simulink model "sim_2dof"  (Simulink 6.2)
settings: Solver=ode45  StartTime=0.0  StopTime=Tmax  MaxStep=0.01*T  RelTol=1e-6
undefined symbols (not defined in the file or in its folder): dF, dG, dK, dKC, dKR, dQ, dQu, dR, k, nF, nG, nK, nKC, nKR, nQ, nQu, nR, T, tauF, tauG, tauQ, tauQu, tauR
settings Model: LastModifiedBy=Administrator
settings OptimizationCC: BlockReduction=off  BooleanDataType=off  InlineInvariantSignals=on
settings HardwareCC: TargetUnknown=on

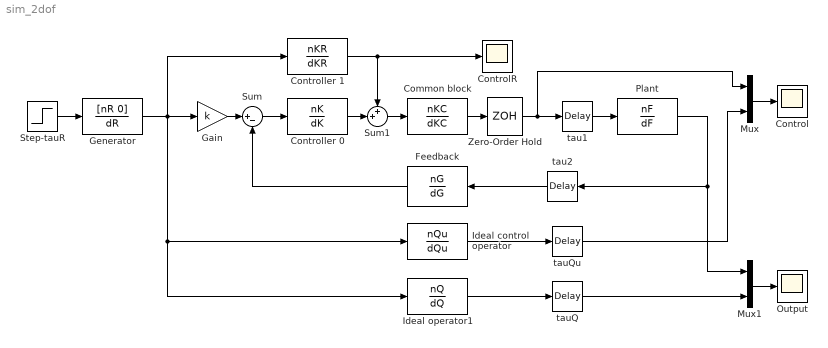
== system sim_2dof ==
  Common block : DiscreteTransferFcn  Numerator=nKC  Denominator=dKC  SampleTime=T
  Control : Scope
      settings: TimeRange=100  YMin=-0.2  YMax=1.2  SaveName=u  DataFormat=Array
  ControlR : Scope
      settings: TimeRange=10  YMin=0  YMax=2.1  SaveName=u1  DataFormat=Array
  Controller 0 : DiscreteTransferFcn  Numerator=nK  Denominator=dK  SampleTime=T
  Controller 1 : DiscreteTransferFcn  Numerator=nKR  Denominator=dKR  SampleTime=T
  Feedback : TransferFcn  Orientation=left  Numerator=nG  Denominator=dG
  Gain : Gain  Gain=k  SaturateOnIntegerOverflow=on
  Generator : TransferFcn  Numerator=[nR 0]  Denominator=dR
  Ideal control operator : TransferFcn  Numerator=nQu  Denominator=dQu
  Ideal operator1 : TransferFcn  Numerator=nQ  Denominator=dQ
  Mux : Mux  Inputs=2
  Mux1 : Mux  Inputs=2
  Output : Scope
      settings: TimeRange=100  YMin=0  YMax=1.4  SaveName=y  DataFormat=Array
  Plant : TransferFcn  Numerator=nF  Denominator=dF
  Step-tauR : Step  Time=tauR
  Sum : Sum  Inputs=|+-  SaturateOnIntegerOverflow=on  InputSameDT=on
  Sum1 : Sum  Inputs=++|  SaturateOnIntegerOverflow=on  InputSameDT=on
  Zero-Order Hold : ZeroOrderHold  SampleTime=T
  tau1 : TransportDelay  DelayTime=tauF  BufferSize=10240
  tau2 : TransportDelay  Orientation=left  DelayTime=tauG  BufferSize=10240
  tauQ : TransportDelay  DelayTime=tauQ  BufferSize=10240
  tauQu : TransportDelay  DelayTime=tauQu  BufferSize=10240
  wires:
  Plant/1 -> Mux1/1, tau2/1
  Step-tauR/1 -> Generator/1
  Mux/1 -> Control/1
  Mux1/1 -> Output/1
  Ideal control operator/1 -> tauQu/1
  tauQu/1 -> Mux/2
  Ideal operator1/1 -> tauQ/1
  tauQ/1 -> Mux1/2
  Controller 0/1 -> Sum1/2
  tau1/1 -> Plant/1
  Sum/1 -> Controller 0/1
  tau2/1 -> Feedback/1
  Feedback/1 -> Sum/2
  Generator/1 -> Ideal operator1/1, Ideal control operator/1, Gain/1, Controller 1/1
  Controller 1/1 -> Sum1/1, ControlR/1
  Zero-Order Hold/1 -> tau1/1, Mux/1
  Sum1/1 -> Common block/1
  Common block/1 -> Zero-Order Hold/1
  Gain/1 -> Sum/1
